simulink model "UPQC_model"  (R2020b)
settings: Solver=FixedStepAuto  StartTime=0.0  StopTime=Tsim  FixedStep=Tsample  MaxStep=Tsample  RelTol=1e-3
values from neighbouring files (symbols this model uses):
  C_parallel_Series = zeros(1,4)    [Netzmodell_Ini_DL.m]    (also in workspace_Ini.mat = [1e-05 1e-05 1e-05 0])
  C_parallel_Shunt = zeros(1,4)    [Netzmodell_Ini_DL.m]    (also in workspace_Ini.mat = [1e-05 1e-05 1e-05 0])
  CC_Ki = 5    [Netzmodell_Ini_DL.m]    (also in workspace_Ini.mat)
  CC_Ki_geg = 5    [Netzmodell_Ini_DL.m]    (also in workspace_Ini.mat)
  CC_Kp = 10    [Netzmodell_Ini_DL.m]    (also in workspace_Ini.mat)
  CC_Kp_geg = 10    [Netzmodell_Ini_DL.m]    (also in workspace_Ini.mat)
  CC_OS =     [workspace_Ini.mat]
  Czk = Szenario.Czk*u    [Netzmodell_Ini_DL.m]    (also in workspace_Ini.mat = 0.003)
  fak_RVC = Szenario.fak_RVC    [Netzmodell_Ini_DL.m]    (also in workspace_Ini.mat = [1 1 1])
  fak_Uns = [1; 1; 1]    [Netzmodell_Ini_DL.m]    (also in workspace_Ini.mat = [1 1 1])
  Flicker_Schaltzeitpunkte_L1 = Schaltzeitpunkte(1,:)    [Netzmodell_Ini_DL.m]    (also in workspace_Ini.mat = 10.5)
  Flicker_Schaltzeitpunkte_L2 = Schaltzeitpunkte(2,:)    [Netzmodell_Ini_DL.m]    (also in workspace_Ini.mat = 10.5)
  Flicker_Schaltzeitpunkte_L3 = Schaltzeitpunkte(3,:)    [Netzmodell_Ini_DL.m]    (also in workspace_Ini.mat = 10.5)
  fs = [f_nom; f_nom; f_nom]    [Netzmodell_Ini_DL.m]    (also in workspace_Ini.mat = [50 50 50])
  fsw = Szenario.fsw*k    [Netzmodell_Ini_DL.m]    (also in workspace_Ini.mat = 20000)
  I_Basis_Ober_L1 = I_Basis_Ober(1)    [Netzmodell_Ini_DL.m]    (also in workspace_Ini.mat = 0)
  I_Basis_Ober_L2 = I_Basis_Ober(2)    [Netzmodell_Ini_DL.m]    (also in workspace_Ini.mat = 0)
  I_Basis_Ober_L3 = I_Basis_Ober(3)    [Netzmodell_Ini_DL.m]    (also in workspace_Ini.mat = 0)
  I_relativ_Ober_L1 = Szenario.I_relativ_Ober_L1    [Netzmodell_Ini_DL.m]    (also in workspace_Ini.mat = [0 100 0 100 100 0 100 100 0 0 0 0 ... (50 elements, 1x50)])
  I_relativ_Ober_L2 = Szenario.I_relativ_Ober_L2    [Netzmodell_Ini_DL.m]    (also in workspace_Ini.mat = [0 100 0 100 100 0 100 100 0 0 0 0 ... (50 elements, 1x50)])
  I_relativ_Ober_L3 = Szenario.I_relativ_Ober_L3    [Netzmodell_Ini_DL.m]    (also in workspace_Ini.mat = [0 100 0 100 100 0 100 100 0 0 0 0 ... (50 elements, 1x50)])
  L_Ausgang_Series = zeros(1,4)    [Netzmodell_Ini_DL.m]    (also in workspace_Ini.mat = [0.00093 0.00093 0.00093 0.00093])
  L_Ausgang_Shunt = zeros(1,4)    [Netzmodell_Ini_DL.m]    (also in workspace_Ini.mat = [0.00093 0.00093 0.00093 0.00093])
  L_Eingang_Series = zeros(1,4)    [Netzmodell_Ini_DL.m]    (also in workspace_Ini.mat = [0.00085 0.00085 0.00085 0.00085])
  L_Eingang_Shunt = zeros(1,4)    [Netzmodell_Ini_DL.m]    (also in workspace_Ini.mat = [0.00085 0.00085 0.00085 0.00085])
  Ls_in = 52.2*u/10    (= 5.22e-06)    [Netzmodell_Ini_DL.m]    (also in workspace_Ini.mat)
  Ltrans = Szenario.Ltrans*m    [Netzmodell_Ini_DL.m]    (also in workspace_Ini.mat = 0.000256)
  OS_off = 6    [Netzmodell_Ini_DL.m]    (also in workspace_Ini.mat)
  OS_on = 1    [Netzmodell_Ini_DL.m]    (also in workspace_Ini.mat)
  Phi_Ober_L1 = Phi_Ober(1)    [Netzmodell_Ini_DL.m]    (also in workspace_Ini.mat = 0)
  Phi_Ober_L2 = Phi_Ober(2)    [Netzmodell_Ini_DL.m]    (also in workspace_Ini.mat = -120)
  Phi_Ober_L3 = Phi_Ober(3)    [Netzmodell_Ini_DL.m]    (also in workspace_Ini.mat = 120)
  Phis = [0; -120; 120]    [Netzmodell_Ini_DL.m]    (also in workspace_Ini.mat = [0 -120 120])
  Pl_Flicker = Pl_Flicker*k    [Netzmodell_Ini_DL.m]    (also in workspace_Ini.mat = [5000 5000 5000])
  Pl_Grund = Szenario.Pl_Grund *k    [Netzmodell_Ini_DL.m]    (also in workspace_Ini.mat = [5 5 5])
  Pl_RVC = Pl_RVC*k    [Netzmodell_Ini_DL.m]    (also in workspace_Ini.mat = [10000 10000 10000])
  Pl_Uns = Pl_Uns*k    [Netzmodell_Ini_DL.m]    (also in workspace_Ini.mat = [25000 10 10])
  Ql_ind_Flicker = Ql_ind_Flicker*k    [Netzmodell_Ini_DL.m]    (also in workspace_Ini.mat = [0 0 0])
  Ql_ind_Grund = Szenario.Ql_ind_Grund*k    [Netzmodell_Ini_DL.m]    (also in workspace_Ini.mat = [0 0 0])
  Ql_ind_RVC = Szenario.Ql_ind_RVC*k    [Netzmodell_Ini_DL.m]    (also in workspace_Ini.mat = [0 0 0])
  Ql_ind_Uns = Ql_ind_Uns*k    [Netzmodell_Ini_DL.m]    (also in workspace_Ini.mat = [0 0 0])
  Ql_kap_Flicker = Ql_kap_Flicker*k    [Netzmodell_Ini_DL.m]    (also in workspace_Ini.mat = [0 0 0])
  Ql_kap_Grund = Szenario.Ql_kap_Grund*k    [Netzmodell_Ini_DL.m]    (also in workspace_Ini.mat = [0 0 0])
  Ql_kap_RVC = Szenario.Ql_kap_RVC*k    [Netzmodell_Ini_DL.m]    (also in workspace_Ini.mat = [0 0 0])
  Ql_kap_Uns = Ql_kap_Uns*k    [Netzmodell_Ini_DL.m]    (also in workspace_Ini.mat = [0 0 0])
  R_Ausgang_Series = zeros(1,4)    [Netzmodell_Ini_DL.m]    (also in workspace_Ini.mat = [0.1 0.1 0.1 0.1])
  R_Ausgang_Shunt = zeros(1,4)    [Netzmodell_Ini_DL.m]    (also in workspace_Ini.mat = [0.1 0.1 0.1 0.1])
  R_Eingang_Series = zeros(1,4)    [Netzmodell_Ini_DL.m]    (also in workspace_Ini.mat = [0.1 0.1 0.1 0.1])
  R_Eingang_Shunt = zeros(1,4)    [Netzmodell_Ini_DL.m]    (also in workspace_Ini.mat = [0.1 0.1 0.1 0.1])
  R_parallel_Series = zeros(1,4)    [Netzmodell_Ini_DL.m]    (also in workspace_Ini.mat = [13 13 13 0])
  R_parallel_Shunt = zeros(1,4)    [Netzmodell_Ini_DL.m]    (also in workspace_Ini.mat = [13 13 13 0])
  R_ZK_Belastung = 20    [Netzmodell_Ini_DL.m]    (also in workspace_Ini.mat)
  Rs_in = 5.2*m/10    (= 0.00052)    [Netzmodell_Ini_DL.m]    (also in workspace_Ini.mat)
  Rtrans = Szenario.Rtrans    [Netzmodell_Ini_DL.m]    (also in workspace_Ini.mat = 0.206)
  RVC_L1_on_off_Zeitpunkte = Szenario.RVC_L1_on_off_Zeitpunkte    [Netzmodell_Ini_DL.m]    (also in workspace_Ini.mat = [10.5 40 10 11 12 13 14 15])
  RVC_L2_on_off_Zeitpunkte = Szenario.RVC_L2_on_off_Zeitpunkte    [Netzmodell_Ini_DL.m]    (also in workspace_Ini.mat = [10.5 40 10 11 12 13 14 15])
  RVC_L3_on_off_Zeitpunkte = Szenario.RVC_L3_on_off_Zeitpunkte    [Netzmodell_Ini_DL.m]    (also in workspace_Ini.mat = [10.5 40 10 11 12 13 14 15])
  RVC_off = 20.5    [Netzmodell_Ini_DL.m]    (also in workspace_Ini.mat)
  RVC_on = 20    [Netzmodell_Ini_DL.m]    (also in workspace_Ini.mat)
  RVC_val = [0.8,0.8,0.8]    [Netzmodell_Ini_DL.m]    (also in workspace_Ini.mat = [0.8 0.8 0.8])
  strans = Szenario.strans    [Netzmodell_Ini_DL.m]    (also in workspace_Ini.mat = 0.25)
  t_breaker_series = tacts    [Netzmodell_Ini_DL.m]    (also in workspace_Ini.mat = 0.5)
  tact = Szenario.tact    [Netzmodell_Ini_DL.m]    (also in workspace_Ini.mat = 0.5)
  tact_OS_Regler = Szenario.tact_OS_Regler    [Netzmodell_Ini_DL.m]    (also in workspace_Ini.mat = 0.5)
  tact_QU = 10    [Netzmodell_Ini_DL.m]    (also in workspace_Ini.mat)
  tacts = Szenario.tacts    [Netzmodell_Ini_DL.m]    (also in workspace_Ini.mat = 0.5)
  Tsample = Szenario.Tsample    [Netzmodell_Ini_DL.m]    (also in workspace_Ini.mat = 5e-06)
  Uns_L1_on_off_Zeitpunkte = Szenario.Uns_L1_on_off_Zeitpunkte    [Netzmodell_Ini_DL.m]    (also in workspace_Ini.mat = [1 6 10 11 12 13 14 15])
  Uns_L2_on_off_Zeitpunkte = Szenario.Uns_L2_on_off_Zeitpunkte    [Netzmodell_Ini_DL.m]    (also in workspace_Ini.mat = [10 30 10 11 12 13 14 15])
  Uns_L3_on_off_Zeitpunkte = Szenario.Uns_L3_on_off_Zeitpunkte    [Netzmodell_Ini_DL.m]    (also in workspace_Ini.mat = [10 30 10 11 12 13 14 15])
  Us = [Us_Amp; Us_Amp; Us_Amp]    [Netzmodell_Ini_DL.m]    (also in workspace_Ini.mat = [326.598632371 326.598632371 326.598632371])
  Us_Amp = sqrt(2)*400/sqrt(3)    [Netzmodell_Ini_DL.m]    (also in workspace_Ini.mat = 326.598632371)
  VC_Ki_gegen = 30    [Netzmodell_Ini_DL.m]    (also in workspace_Ini.mat)
  VC_Ki_gegen_shunt = 15    [Netzmodell_Ini_DL.m]    (also in workspace_Ini.mat)
  VC_Ki_mit = 5    [Netzmodell_Ini_DL.m]    (also in workspace_Ini.mat)
  VC_Kp_gegen = 5    [workspace_Ini.mat]
  VC_Kp_gegen_shunt = 2    [Netzmodell_Ini_DL.m]    (also in workspace_Ini.mat)
  VC_Kp_mit = 10    [Netzmodell_Ini_DL.m]    (also in workspace_Ini.mat)
  VC_ZK_Ki = 5    [Netzmodell_Ini_DL.m]    (also in workspace_Ini.mat)
  VC_ZK_Kp = 0.5    [Netzmodell_Ini_DL.m]    (also in workspace_Ini.mat)
  Vielfache_Ober_L1 = Szenario.Vielfache_Ober_L1    [Netzmodell_Ini_DL.m]    (also in workspace_Ini.mat = [1 2 3 4 5 6 7 8 9 10 11 12 ... (50 elements, 1x50)])
  Vielfache_Ober_L2 = Szenario.Vielfache_Ober_L2    [Netzmodell_Ini_DL.m]    (also in workspace_Ini.mat = [1 2 3 4 5 6 7 8 9 10 11 12 ... (50 elements, 1x50)])
  Vielfache_Ober_L3 = Szenario.Vielfache_Ober_L3    [Netzmodell_Ini_DL.m]    (also in workspace_Ini.mat = [1 2 3 4 5 6 7 8 9 10 11 12 ... (50 elements, 1x50)])
  ZK_Belastung_off = 100    [Netzmodell_Ini_DL.m]    (also in workspace_Ini.mat)
  ZK_Belastung_on = 100    [Netzmodell_Ini_DL.m]    (also in workspace_Ini.mat)
  Zwischenkreisspannung = 700    [Netzmodell_Ini_DL.m]    (also in workspace_Ini.mat)
undefined symbols (not defined in the file or in its folder): LAusgang, RReiheL3
libraries: powerlib x221, powerlib_meascontrol x80, pid_lib x23, eeTransforms x4, eePwmGeneratorTwoLevel x2, dspstat3 x1
(part 15 of 16)

== system UPQC_model/Shunt UPQC/Shuntkompensator/dq_Netz/Tdq+1_4 ==
  In1 : Inport
  In2 : Inport  Port=2
  Add : Sum  Inputs=|++
  Add1 : Sum  Inputs=|++
  Cos : Trigonometry  Operator=cos
  Cos1 : Trigonometry  Operator=cos
  Demux : Demux  Outputs=2
  Gain : Gain  Gain=-1
  Mux : Mux  Inputs=2
  Product{,1..3} (4 alike) : Product
  Sin : Trigonometry
  Sin1 : Trigonometry
  Out1 : Outport
  wires:
  Add1/1 -> Mux/2
  Product3/1 -> Add1/2
  [alpha] -> Product2/1
  [alpha] -> Product/1
  Product/1 -> Add/1
  Cos1/1 -> Product3/1
  Sin1/1 -> Gain/1
  [beta] -> Product1/2
  Product1/1 -> Add/2
  Gain/1 -> Product2/2
  Mux/1 -> [dq]
  Add/1 -> Mux/1
  Sin/1 -> Product1/1
  Product2/1 -> Add1/1
  [beta] -> Product3/2
  Cos/1 -> Product/2
  In1/1 -> Demux/1  "vab"
  [dq] -> Out1/1  "dq"
  In2/1 -> [theta]  "theta"
  [theta] -> Sin/1, Cos/1
  [theta] -> Sin1/1, Cos1/1
  Demux/1 -> [alpha]
  Demux/2 -> [beta]

== system UPQC_model/Shunt UPQC/Shuntkompensator/dq_Netz/Tdq+1_5 ==
  In1 : Inport
  In2 : Inport  Port=2
  Add : Sum  Inputs=|++
  Add1 : Sum  Inputs=|++
  Cos : Trigonometry  Operator=cos
  Cos1 : Trigonometry  Operator=cos
  Demux : Demux  Outputs=2
  Gain : Gain  Gain=-1
  Mux : Mux  Inputs=2
  Product{,1..3} (4 alike) : Product
  Sin : Trigonometry
  Sin1 : Trigonometry
  Out1 : Outport
  wires:
  Add1/1 -> Mux/2
  Product3/1 -> Add1/2
  [alpha] -> Product2/1
  [alpha] -> Product/1
  Product/1 -> Add/1
  Cos1/1 -> Product3/1
  Sin1/1 -> Gain/1
  [beta] -> Product1/2
  Product1/1 -> Add/2
  Gain/1 -> Product2/2
  Mux/1 -> [dq]
  Add/1 -> Mux/1
  Sin/1 -> Product1/1
  Product2/1 -> Add1/1
  [beta] -> Product3/2
  Cos/1 -> Product/2
  In1/1 -> Demux/1  "vab"
  [dq] -> Out1/1  "dq"
  In2/1 -> [theta]  "theta"
  [theta] -> Sin/1, Cos/1
  [theta] -> Sin1/1, Cos1/1
  Demux/1 -> [alpha]
  Demux/2 -> [beta]

== system UPQC_model/Shunt UPQC/Shuntkompensator/dq_Netz/Tdq+1_6 ==
  In1 : Inport
  In2 : Inport  Port=2
  Add : Sum  Inputs=|++
  Add1 : Sum  Inputs=|++
  Cos : Trigonometry  Operator=cos
  Cos1 : Trigonometry  Operator=cos
  Demux : Demux  Outputs=2
  Gain : Gain  Gain=-1
  Mux : Mux  Inputs=2
  Product{,1..3} (4 alike) : Product
  Sin : Trigonometry
  Sin1 : Trigonometry
  Out1 : Outport
  wires:
  Demux/2 -> [beta]
  Demux/1 -> [alpha]
  [theta] -> Cos1/1, Sin1/1
  [theta] -> Cos/1, Sin/1
  In2/1 -> [theta]  "theta"
  [dq] -> Out1/1  "dq"
  In1/1 -> Demux/1  "vab"
  Cos/1 -> Product/2
  [beta] -> Product3/2
  Product2/1 -> Add1/1
  Sin/1 -> Product1/1
  Add/1 -> Mux/1
  Mux/1 -> [dq]
  Gain/1 -> Product2/2
  Product1/1 -> Add/2
  [beta] -> Product1/2
  Sin1/1 -> Gain/1
  Cos1/1 -> Product3/1
  Product/1 -> Add/1
  [alpha] -> Product/1
  [alpha] -> Product2/1
  Product3/1 -> Add1/2
  Add1/1 -> Mux/2

== system UPQC_model/Shunt UPQC/Shuntkompensator/dq_Netz/Tdq+1_7 ==
  In1 : Inport
  In2 : Inport  Port=2
  Add : Sum  Inputs=|++
  Add1 : Sum  Inputs=|++
  Cos : Trigonometry  Operator=cos
  Cos1 : Trigonometry  Operator=cos
  Demux : Demux  Outputs=2
  Gain : Gain  Gain=-1
  Mux : Mux  Inputs=2
  Product{,1..3} (4 alike) : Product
  Sin : Trigonometry
  Sin1 : Trigonometry
  Out1 : Outport
  wires:
  Add1/1 -> Mux/2
  Product3/1 -> Add1/2
  [alpha] -> Product2/1
  [alpha] -> Product/1
  Product/1 -> Add/1
  Cos1/1 -> Product3/1
  Sin1/1 -> Gain/1
  [beta] -> Product1/2
  Product1/1 -> Add/2
  Gain/1 -> Product2/2
  Mux/1 -> [dq]
  Add/1 -> Mux/1
  Sin/1 -> Product1/1
  Product2/1 -> Add1/1
  [beta] -> Product3/2
  Cos/1 -> Product/2
  In1/1 -> Demux/1  "vab"
  [dq] -> Out1/1  "dq"
  In2/1 -> [theta]  "theta"
  [theta] -> Sin/1, Cos/1
  [theta] -> Sin1/1, Cos1/1
  Demux/1 -> [alpha]
  Demux/2 -> [beta]

== system UPQC_model/Shunt UPQC/Shuntkompensator/dq_Netz/Tdq+1_8 ==
  In1 : Inport
  In2 : Inport  Port=2
  Add : Sum  Inputs=|++
  Add1 : Sum  Inputs=|++
  Cos : Trigonometry  Operator=cos
  Cos1 : Trigonometry  Operator=cos
  Demux : Demux  Outputs=2
  Gain : Gain  Gain=-1
  Mux : Mux  Inputs=2
  Product{,1..3} (4 alike) : Product
  Sin : Trigonometry
  Sin1 : Trigonometry
  Out1 : Outport
  wires:
  Demux/2 -> [beta]
  Demux/1 -> [alpha]
  [theta] -> Cos1/1, Sin1/1
  [theta] -> Cos/1, Sin/1
  In2/1 -> [theta]  "theta"
  [dq] -> Out1/1  "dq"
  In1/1 -> Demux/1  "vab"
  Cos/1 -> Product/2
  [beta] -> Product3/2
  Product2/1 -> Add1/1
  Sin/1 -> Product1/1
  Add/1 -> Mux/1
  Mux/1 -> [dq]
  Gain/1 -> Product2/2
  Product1/1 -> Add/2
  [beta] -> Product1/2
  Sin1/1 -> Gain/1
  Cos1/1 -> Product3/1
  Product/1 -> Add/1
  [alpha] -> Product/1
  [alpha] -> Product2/1
  Product3/1 -> Add1/2
  Add1/1 -> Mux/2

== system UPQC_model/Shunt UPQC/Shuntkompensator/dq_Shunt/Entkopplungszelle1 ==
  In3 : Inport
  In4 : Inport  Port=2
  In1 : Inport  Port=3
  Add : Sum  Inputs=|+-
  Add1 : Sum  Inputs=|+-
  Add2 : Sum  Inputs=|++
  Add3 : Sum  Inputs=|+-
  Cos : Trigonometry  Operator=cos
  Demux : Demux  Outputs=2
  Demux1 : Demux  Outputs=2
  Mux : Mux  Inputs=2
  Product{,1..3} (4 alike) : Product
  Sin : Trigonometry
  Out2 : Outport
  wires:
  Mux/1 -> Out2/1
  Demux1/1 -> Product1/1, Product/2  "d"
  In1/1 -> Demux1/1  "dq"
  In4/1 -> Sin/1, Cos/1  "theta"
  Add3/1 -> Mux/2
  Add1/1 -> Mux/1
  Product1/1 -> Add2/2
  Product2/1 -> Add3/2
  In3/1 -> Demux/1  "vdqmit"
  Sin/1 -> Product1/2, Product3/1
  Cos/1 -> Product2/2, Product/1
  Add/1 -> Add1/1
  Demux/2 -> Add2/1
  Product3/1 -> Add1/2
  Add2/1 -> Add3/1
  Demux/1 -> Add/1
  Demux1/2 -> Product3/2, Product2/1  "q"
  Product/1 -> Add/2

== system UPQC_model/Shunt UPQC/Shuntkompensator/dq_Shunt/Entkopplungszelle10 ==
  In3 : Inport
  In4 : Inport  Port=2
  In1 : Inport  Port=3
  Add : Sum  Inputs=|+-
  Add1 : Sum  Inputs=|+-
  Add2 : Sum  Inputs=|++
  Add3 : Sum  Inputs=|+-
  Cos : Trigonometry  Operator=cos
  Demux : Demux  Outputs=2
  Demux1 : Demux  Outputs=2
  Mux : Mux  Inputs=2
  Product{,1..3} (4 alike) : Product
  Sin : Trigonometry
  Out2 : Outport
  wires:
  Mux/1 -> Out2/1
  Demux1/1 -> Product1/1, Product/2  "d"
  In1/1 -> Demux1/1  "dq"
  In4/1 -> Sin/1, Cos/1  "theta"
  Add3/1 -> Mux/2
  Add1/1 -> Mux/1
  Product1/1 -> Add2/2
  Product2/1 -> Add3/2
  In3/1 -> Demux/1  "vdqmit"
  Sin/1 -> Product1/2, Product3/1
  Cos/1 -> Product2/2, Product/1
  Add/1 -> Add1/1
  Demux/2 -> Add2/1
  Product3/1 -> Add1/2
  Add2/1 -> Add3/1
  Demux/1 -> Add/1
  Demux1/2 -> Product3/2, Product2/1  "q"
  Product/1 -> Add/2

== system UPQC_model/Shunt UPQC/Shuntkompensator/dq_Shunt/Entkopplungszelle11 ==
  In3 : Inport
  In4 : Inport  Port=2
  In1 : Inport  Port=3
  Add : Sum  Inputs=|+-
  Add1 : Sum  Inputs=|+-
  Add2 : Sum  Inputs=|++
  Add3 : Sum  Inputs=|+-
  Cos : Trigonometry  Operator=cos
  Demux : Demux  Outputs=2
  Demux1 : Demux  Outputs=2
  Mux : Mux  Inputs=2
  Product{,1..3} (4 alike) : Product
  Sin : Trigonometry
  Out2 : Outport
  wires:
  Mux/1 -> Out2/1
  Demux1/1 -> Product1/1, Product/2  "d"
  In1/1 -> Demux1/1  "dq"
  In4/1 -> Sin/1, Cos/1  "theta"
  Add3/1 -> Mux/2
  Add1/1 -> Mux/1
  Product1/1 -> Add2/2
  Product2/1 -> Add3/2
  In3/1 -> Demux/1  "vdqmit"
  Sin/1 -> Product1/2, Product3/1
  Cos/1 -> Product2/2, Product/1
  Add/1 -> Add1/1
  Demux/2 -> Add2/1
  Product3/1 -> Add1/2
  Add2/1 -> Add3/1
  Demux/1 -> Add/1
  Demux1/2 -> Product3/2, Product2/1  "q"
  Product/1 -> Add/2

== system UPQC_model/Shunt UPQC/Shuntkompensator/dq_Shunt/Entkopplungszelle12 ==
  In3 : Inport
  In4 : Inport  Port=2
  In1 : Inport  Port=3
  Add : Sum  Inputs=|+-
  Add1 : Sum  Inputs=|+-
  Add2 : Sum  Inputs=|++
  Add3 : Sum  Inputs=|+-
  Cos : Trigonometry  Operator=cos
  Demux : Demux  Outputs=2
  Demux1 : Demux  Outputs=2
  Mux : Mux  Inputs=2
  Product{,1..3} (4 alike) : Product
  Sin : Trigonometry
  Out2 : Outport
  wires:
  Mux/1 -> Out2/1
  Demux1/1 -> Product1/1, Product/2  "d"
  In1/1 -> Demux1/1  "dq"
  In4/1 -> Sin/1, Cos/1  "theta"
  Add3/1 -> Mux/2
  Add1/1 -> Mux/1
  Product1/1 -> Add2/2
  Product2/1 -> Add3/2
  In3/1 -> Demux/1  "vdqmit"
  Sin/1 -> Product1/2, Product3/1
  Cos/1 -> Product2/2, Product/1
  Add/1 -> Add1/1
  Demux/2 -> Add2/1
  Product3/1 -> Add1/2
  Add2/1 -> Add3/1
  Demux/1 -> Add/1
  Demux1/2 -> Product3/2, Product2/1  "q"
  Product/1 -> Add/2

== system UPQC_model/Shunt UPQC/Shuntkompensator/dq_Shunt/Entkopplungszelle13 ==
  In3 : Inport
  In4 : Inport  Port=2
  In1 : Inport  Port=3
  Add : Sum  Inputs=|+-
  Add1 : Sum  Inputs=|+-
  Add2 : Sum  Inputs=|++
  Add3 : Sum  Inputs=|+-
  Cos : Trigonometry  Operator=cos
  Demux : Demux  Outputs=2
  Demux1 : Demux  Outputs=2
  Mux : Mux  Inputs=2
  Product{,1..3} (4 alike) : Product
  Sin : Trigonometry
  Out2 : Outport
  wires:
  Mux/1 -> Out2/1
  Demux1/1 -> Product1/1, Product/2  "d"
  In1/1 -> Demux1/1  "dq"
  In4/1 -> Sin/1, Cos/1  "theta"
  Add3/1 -> Mux/2
  Add1/1 -> Mux/1
  Product1/1 -> Add2/2
  Product2/1 -> Add3/2
  In3/1 -> Demux/1  "vdqmit"
  Sin/1 -> Product1/2, Product3/1
  Cos/1 -> Product2/2, Product/1
  Add/1 -> Add1/1
  Demux/2 -> Add2/1
  Product3/1 -> Add1/2
  Add2/1 -> Add3/1
  Demux/1 -> Add/1
  Demux1/2 -> Product3/2, Product2/1  "q"
  Product/1 -> Add/2

== system UPQC_model/Shunt UPQC/Shuntkompensator/dq_Shunt/Entkopplungszelle14 ==
  In3 : Inport
  In4 : Inport  Port=2
  In1 : Inport  Port=3
  Add : Sum  Inputs=|+-
  Add1 : Sum  Inputs=|+-
  Add2 : Sum  Inputs=|++
  Add3 : Sum  Inputs=|+-
  Cos : Trigonometry  Operator=cos
  Demux : Demux  Outputs=2
  Demux1 : Demux  Outputs=2
  Mux : Mux  Inputs=2
  Product{,1..3} (4 alike) : Product
  Sin : Trigonometry
  Out2 : Outport
  wires:
  Mux/1 -> Out2/1
  Demux1/1 -> Product1/1, Product/2  "d"
  In1/1 -> Demux1/1  "dq"
  In4/1 -> Sin/1, Cos/1  "theta"
  Add3/1 -> Mux/2
  Add1/1 -> Mux/1
  Product1/1 -> Add2/2
  Product2/1 -> Add3/2
  In3/1 -> Demux/1  "vdqmit"
  Sin/1 -> Product1/2, Product3/1
  Cos/1 -> Product2/2, Product/1
  Add/1 -> Add1/1
  Demux/2 -> Add2/1
  Product3/1 -> Add1/2
  Add2/1 -> Add3/1
  Demux/1 -> Add/1
  Demux1/2 -> Product3/2, Product2/1  "q"
  Product/1 -> Add/2

== system UPQC_model/Shunt UPQC/Shuntkompensator/dq_Shunt/Entkopplungszelle15 ==
  In3 : Inport
  In4 : Inport  Port=2
  In1 : Inport  Port=3
  Add : Sum  Inputs=|+-
  Add1 : Sum  Inputs=|+-
  Add2 : Sum  Inputs=|++
  Add3 : Sum  Inputs=|+-
  Cos : Trigonometry  Operator=cos
  Demux : Demux  Outputs=2
  Demux1 : Demux  Outputs=2
  Mux : Mux  Inputs=2
  Product{,1..3} (4 alike) : Product
  Sin : Trigonometry
  Out2 : Outport
  wires:
  Product/1 -> Add/2
  Demux1/2 -> Product2/1, Product3/2  "q"
  Demux/1 -> Add/1
  Add2/1 -> Add3/1
  Product3/1 -> Add1/2
  Demux/2 -> Add2/1
  Add/1 -> Add1/1
  Cos/1 -> Product/1, Product2/2
  Sin/1 -> Product3/1, Product1/2
  In3/1 -> Demux/1  "vdqmit"
  Product2/1 -> Add3/2
  Product1/1 -> Add2/2
  Add1/1 -> Mux/1
  Add3/1 -> Mux/2
  In4/1 -> Cos/1, Sin/1  "theta"
  In1/1 -> Demux1/1  "dq"
  Demux1/1 -> Product/2, Product1/1  "d"
  Mux/1 -> Out2/1

== system UPQC_model/Shunt UPQC/Shuntkompensator/dq_Shunt/Entkopplungszelle16 ==
  In3 : Inport
  In4 : Inport  Port=2
  In1 : Inport  Port=3
  Add : Sum  Inputs=|+-
  Add1 : Sum  Inputs=|+-
  Add2 : Sum  Inputs=|++
  Add3 : Sum  Inputs=|+-
  Cos : Trigonometry  Operator=cos
  Demux : Demux  Outputs=2
  Demux1 : Demux  Outputs=2
  Mux : Mux  Inputs=2
  Product{,1..3} (4 alike) : Product
  Sin : Trigonometry
  Out2 : Outport
  wires:
  Mux/1 -> Out2/1
  Demux1/1 -> Product1/1, Product/2  "d"
  In1/1 -> Demux1/1  "dq"
  In4/1 -> Sin/1, Cos/1  "theta"
  Add3/1 -> Mux/2
  Add1/1 -> Mux/1
  Product1/1 -> Add2/2
  Product2/1 -> Add3/2
  In3/1 -> Demux/1  "vdqmit"
  Sin/1 -> Product1/2, Product3/1
  Cos/1 -> Product2/2, Product/1
  Add/1 -> Add1/1
  Demux/2 -> Add2/1
  Product3/1 -> Add1/2
  Add2/1 -> Add3/1
  Demux/1 -> Add/1
  Demux1/2 -> Product3/2, Product2/1  "q"
  Product/1 -> Add/2

== system UPQC_model/Shunt UPQC/Shuntkompensator/dq_Shunt/Entkopplungszelle17 ==
  In3 : Inport
  In4 : Inport  Port=2
  In1 : Inport  Port=3
  Add : Sum  Inputs=|+-
  Add1 : Sum  Inputs=|+-
  Add2 : Sum  Inputs=|++
  Add3 : Sum  Inputs=|+-
  Cos : Trigonometry  Operator=cos
  Demux : Demux  Outputs=2
  Demux1 : Demux  Outputs=2
  Mux : Mux  Inputs=2
  Product{,1..3} (4 alike) : Product
  Sin : Trigonometry
  Out2 : Outport
  wires:
  Product/1 -> Add/2
  Demux1/2 -> Product2/1, Product3/2  "q"
  Demux/1 -> Add/1
  Add2/1 -> Add3/1
  Product3/1 -> Add1/2
  Demux/2 -> Add2/1
  Add/1 -> Add1/1
  Cos/1 -> Product/1, Product2/2
  Sin/1 -> Product3/1, Product1/2
  In3/1 -> Demux/1  "vdqmit"
  Product2/1 -> Add3/2
  Product1/1 -> Add2/2
  Add1/1 -> Mux/1
  Add3/1 -> Mux/2
  In4/1 -> Cos/1, Sin/1  "theta"
  In1/1 -> Demux1/1  "dq"
  Demux1/1 -> Product/2, Product1/1  "d"
  Mux/1 -> Out2/1

== system UPQC_model/Shunt UPQC/Shuntkompensator/dq_Shunt/Entkopplungszelle18 ==
  In3 : Inport
  In4 : Inport  Port=2
  In1 : Inport  Port=3
  Add : Sum  Inputs=|+-
  Add1 : Sum  Inputs=|+-
  Add2 : Sum  Inputs=|++
  Add3 : Sum  Inputs=|+-
  Cos : Trigonometry  Operator=cos
  Demux : Demux  Outputs=2
  Demux1 : Demux  Outputs=2
  Mux : Mux  Inputs=2
  Product{,1..3} (4 alike) : Product
  Sin : Trigonometry
  Out2 : Outport
  wires:
  Mux/1 -> Out2/1
  Demux1/1 -> Product1/1, Product/2  "d"
  In1/1 -> Demux1/1  "dq"
  In4/1 -> Sin/1, Cos/1  "theta"
  Add3/1 -> Mux/2
  Add1/1 -> Mux/1
  Product1/1 -> Add2/2
  Product2/1 -> Add3/2
  In3/1 -> Demux/1  "vdqmit"
  Sin/1 -> Product1/2, Product3/1
  Cos/1 -> Product2/2, Product/1
  Add/1 -> Add1/1
  Demux/2 -> Add2/1
  Product3/1 -> Add1/2
  Add2/1 -> Add3/1
  Demux/1 -> Add/1
  Demux1/2 -> Product3/2, Product2/1  "q"
  Product/1 -> Add/2

== system UPQC_model/Shunt UPQC/Shuntkompensator/dq_Shunt/Entkopplungszelle19 ==
  In3 : Inport
  In4 : Inport  Port=2
  In1 : Inport  Port=3
  Add : Sum  Inputs=|+-
  Add1 : Sum  Inputs=|+-
  Add2 : Sum  Inputs=|++
  Add3 : Sum  Inputs=|+-
  Cos : Trigonometry  Operator=cos
  Demux : Demux  Outputs=2
  Demux1 : Demux  Outputs=2
  Mux : Mux  Inputs=2
  Product{,1..3} (4 alike) : Product
  Sin : Trigonometry
  Out2 : Outport
  wires:
  Product/1 -> Add/2
  Demux1/2 -> Product2/1, Product3/2  "q"
  Demux/1 -> Add/1
  Add2/1 -> Add3/1
  Product3/1 -> Add1/2
  Demux/2 -> Add2/1
  Add/1 -> Add1/1
  Cos/1 -> Product/1, Product2/2
  Sin/1 -> Product3/1, Product1/2
  In3/1 -> Demux/1  "vdqmit"
  Product2/1 -> Add3/2
  Product1/1 -> Add2/2
  Add1/1 -> Mux/1
  Add3/1 -> Mux/2
  In4/1 -> Cos/1, Sin/1  "theta"
  In1/1 -> Demux1/1  "dq"
  Demux1/1 -> Product/2, Product1/1  "d"
  Mux/1 -> Out2/1

== system UPQC_model/Shunt UPQC/Shuntkompensator/dq_Shunt/Entkopplungszelle2 ==
  In3 : Inport
  In4 : Inport  Port=2
  In1 : Inport  Port=3
  Add : Sum  Inputs=|+-
  Add1 : Sum  Inputs=|+-
  Add2 : Sum  Inputs=|++
  Add3 : Sum  Inputs=|+-
  Cos : Trigonometry  Operator=cos
  Demux : Demux  Outputs=2
  Demux1 : Demux  Outputs=2
  Mux : Mux  Inputs=2
  Product{,1..3} (4 alike) : Product
  Sin : Trigonometry
  Out2 : Outport
  wires:
  Mux/1 -> Out2/1
  Demux1/1 -> Product1/1, Product/2  "d"
  In1/1 -> Demux1/1  "dq"
  In4/1 -> Sin/1, Cos/1  "theta"
  Add3/1 -> Mux/2
  Add1/1 -> Mux/1
  Product1/1 -> Add2/2
  Product2/1 -> Add3/2
  In3/1 -> Demux/1  "vdqmit"
  Sin/1 -> Product1/2, Product3/1
  Cos/1 -> Product2/2, Product/1
  Add/1 -> Add1/1
  Demux/2 -> Add2/1
  Product3/1 -> Add1/2
  Add2/1 -> Add3/1
  Demux/1 -> Add/1
  Demux1/2 -> Product3/2, Product2/1  "q"
  Product/1 -> Add/2

== system UPQC_model/Shunt UPQC/Shuntkompensator/dq_Shunt/Entkopplungszelle20 ==
  In3 : Inport
  In4 : Inport  Port=2
  In1 : Inport  Port=3
  Add : Sum  Inputs=|+-
  Add1 : Sum  Inputs=|+-
  Add2 : Sum  Inputs=|++
  Add3 : Sum  Inputs=|+-
  Cos : Trigonometry  Operator=cos
  Demux : Demux  Outputs=2
  Demux1 : Demux  Outputs=2
  Mux : Mux  Inputs=2
  Product{,1..3} (4 alike) : Product
  Sin : Trigonometry
  Out2 : Outport
  wires:
  Mux/1 -> Out2/1
  Demux1/1 -> Product1/1, Product/2  "d"
  In1/1 -> Demux1/1  "dq"
  In4/1 -> Sin/1, Cos/1  "theta"
  Add3/1 -> Mux/2
  Add1/1 -> Mux/1
  Product1/1 -> Add2/2
  Product2/1 -> Add3/2
  In3/1 -> Demux/1  "vdqmit"
  Sin/1 -> Product1/2, Product3/1
  Cos/1 -> Product2/2, Product/1
  Add/1 -> Add1/1
  Demux/2 -> Add2/1
  Product3/1 -> Add1/2
  Add2/1 -> Add3/1
  Demux/1 -> Add/1
  Demux1/2 -> Product3/2, Product2/1  "q"
  Product/1 -> Add/2

== system UPQC_model/Shunt UPQC/Shuntkompensator/dq_Shunt/Entkopplungszelle21 ==
  In3 : Inport
  In4 : Inport  Port=2
  In1 : Inport  Port=3
  Add : Sum  Inputs=|+-
  Add1 : Sum  Inputs=|+-
  Add2 : Sum  Inputs=|++
  Add3 : Sum  Inputs=|+-
  Cos : Trigonometry  Operator=cos
  Demux : Demux  Outputs=2
  Demux1 : Demux  Outputs=2
  Mux : Mux  Inputs=2
  Product{,1..3} (4 alike) : Product
  Sin : Trigonometry
  Out2 : Outport
  wires:
  Product/1 -> Add/2
  Demux1/2 -> Product2/1, Product3/2  "q"
  Demux/1 -> Add/1
  Add2/1 -> Add3/1
  Product3/1 -> Add1/2
  Demux/2 -> Add2/1
  Add/1 -> Add1/1
  Cos/1 -> Product/1, Product2/2
  Sin/1 -> Product3/1, Product1/2
  In3/1 -> Demux/1  "vdqmit"
  Product2/1 -> Add3/2
  Product1/1 -> Add2/2
  Add1/1 -> Mux/1
  Add3/1 -> Mux/2
  In4/1 -> Cos/1, Sin/1  "theta"
  In1/1 -> Demux1/1  "dq"
  Demux1/1 -> Product/2, Product1/1  "d"
  Mux/1 -> Out2/1

== system UPQC_model/Shunt UPQC/Shuntkompensator/dq_Shunt/Entkopplungszelle22 ==
  In3 : Inport
  In4 : Inport  Port=2
  In1 : Inport  Port=3
  Add : Sum  Inputs=|+-
  Add1 : Sum  Inputs=|+-
  Add2 : Sum  Inputs=|++
  Add3 : Sum  Inputs=|+-
  Cos : Trigonometry  Operator=cos
  Demux : Demux  Outputs=2
  Demux1 : Demux  Outputs=2
  Mux : Mux  Inputs=2
  Product{,1..3} (4 alike) : Product
  Sin : Trigonometry
  Out2 : Outport
  wires:
  Mux/1 -> Out2/1
  Demux1/1 -> Product1/1, Product/2  "d"
  In1/1 -> Demux1/1  "dq"
  In4/1 -> Sin/1, Cos/1  "theta"
  Add3/1 -> Mux/2
  Add1/1 -> Mux/1
  Product1/1 -> Add2/2
  Product2/1 -> Add3/2
  In3/1 -> Demux/1  "vdqmit"
  Sin/1 -> Product1/2, Product3/1
  Cos/1 -> Product2/2, Product/1
  Add/1 -> Add1/1
  Demux/2 -> Add2/1
  Product3/1 -> Add1/2
  Add2/1 -> Add3/1
  Demux/1 -> Add/1
  Demux1/2 -> Product3/2, Product2/1  "q"
  Product/1 -> Add/2

== system UPQC_model/Shunt UPQC/Shuntkompensator/dq_Shunt/Entkopplungszelle23 ==
  In3 : Inport
  In4 : Inport  Port=2
  In1 : Inport  Port=3
  Add : Sum  Inputs=|+-
  Add1 : Sum  Inputs=|+-
  Add2 : Sum  Inputs=|++
  Add3 : Sum  Inputs=|+-
  Cos : Trigonometry  Operator=cos
  Demux : Demux  Outputs=2
  Demux1 : Demux  Outputs=2
  Mux : Mux  Inputs=2
  Product{,1..3} (4 alike) : Product
  Sin : Trigonometry
  Out2 : Outport
  wires:
  Product/1 -> Add/2
  Demux1/2 -> Product2/1, Product3/2  "q"
  Demux/1 -> Add/1
  Add2/1 -> Add3/1
  Product3/1 -> Add1/2
  Demux/2 -> Add2/1
  Add/1 -> Add1/1
  Cos/1 -> Product/1, Product2/2
  Sin/1 -> Product3/1, Product1/2
  In3/1 -> Demux/1  "vdqmit"
  Product2/1 -> Add3/2
  Product1/1 -> Add2/2
  Add1/1 -> Mux/1
  Add3/1 -> Mux/2
  In4/1 -> Cos/1, Sin/1  "theta"
  In1/1 -> Demux1/1  "dq"
  Demux1/1 -> Product/2, Product1/1  "d"
  Mux/1 -> Out2/1

== system UPQC_model/Shunt UPQC/Shuntkompensator/dq_Shunt/Entkopplungszelle24 ==
  In3 : Inport
  In4 : Inport  Port=2
  In1 : Inport  Port=3
  Add : Sum  Inputs=|+-
  Add1 : Sum  Inputs=|+-
  Add2 : Sum  Inputs=|++
  Add3 : Sum  Inputs=|+-
  Cos : Trigonometry  Operator=cos
  Demux : Demux  Outputs=2
  Demux1 : Demux  Outputs=2
  Mux : Mux  Inputs=2
  Product{,1..3} (4 alike) : Product
  Sin : Trigonometry
  Out2 : Outport
  wires:
  Mux/1 -> Out2/1
  Demux1/1 -> Product1/1, Product/2  "d"
  In1/1 -> Demux1/1  "dq"
  In4/1 -> Sin/1, Cos/1  "theta"
  Add3/1 -> Mux/2
  Add1/1 -> Mux/1
  Product1/1 -> Add2/2
  Product2/1 -> Add3/2
  In3/1 -> Demux/1  "vdqmit"
  Sin/1 -> Product1/2, Product3/1
  Cos/1 -> Product2/2, Product/1
  Add/1 -> Add1/1
  Demux/2 -> Add2/1
  Product3/1 -> Add1/2
  Add2/1 -> Add3/1
  Demux/1 -> Add/1
  Demux1/2 -> Product3/2, Product2/1  "q"
  Product/1 -> Add/2

== system UPQC_model/Shunt UPQC/Shuntkompensator/dq_Shunt/Entkopplungszelle25 ==
  In3 : Inport
  In4 : Inport  Port=2
  In1 : Inport  Port=3
  Add : Sum  Inputs=|+-
  Add1 : Sum  Inputs=|+-
  Add2 : Sum  Inputs=|++
  Add3 : Sum  Inputs=|+-
  Cos : Trigonometry  Operator=cos
  Demux : Demux  Outputs=2
  Demux1 : Demux  Outputs=2
  Mux : Mux  Inputs=2
  Product{,1..3} (4 alike) : Product
  Sin : Trigonometry
  Out2 : Outport
  wires:
  Product/1 -> Add/2
  Demux1/2 -> Product2/1, Product3/2  "q"
  Demux/1 -> Add/1
  Add2/1 -> Add3/1
  Product3/1 -> Add1/2
  Demux/2 -> Add2/1
  Add/1 -> Add1/1
  Cos/1 -> Product/1, Product2/2
  Sin/1 -> Product3/1, Product1/2
  In3/1 -> Demux/1  "vdqmit"
  Product2/1 -> Add3/2
  Product1/1 -> Add2/2
  Add1/1 -> Mux/1
  Add3/1 -> Mux/2
  In4/1 -> Cos/1, Sin/1  "theta"
  In1/1 -> Demux1/1  "dq"
  Demux1/1 -> Product/2, Product1/1  "d"
  Mux/1 -> Out2/1

== system UPQC_model/Shunt UPQC/Shuntkompensator/dq_Shunt/Entkopplungszelle26 ==
  In3 : Inport
  In4 : Inport  Port=2
  In1 : Inport  Port=3
  Add : Sum  Inputs=|+-
  Add1 : Sum  Inputs=|+-
  Add2 : Sum  Inputs=|++
  Add3 : Sum  Inputs=|+-
  Cos : Trigonometry  Operator=cos
  Demux : Demux  Outputs=2
  Demux1 : Demux  Outputs=2
  Mux : Mux  Inputs=2
  Product{,1..3} (4 alike) : Product
  Sin : Trigonometry
  Out2 : Outport
  wires:
  Mux/1 -> Out2/1
  Demux1/1 -> Product1/1, Product/2  "d"
  In1/1 -> Demux1/1  "dq"
  In4/1 -> Sin/1, Cos/1  "theta"
  Add3/1 -> Mux/2
  Add1/1 -> Mux/1
  Product1/1 -> Add2/2
  Product2/1 -> Add3/2
  In3/1 -> Demux/1  "vdqmit"
  Sin/1 -> Product1/2, Product3/1
  Cos/1 -> Product2/2, Product/1
  Add/1 -> Add1/1
  Demux/2 -> Add2/1
  Product3/1 -> Add1/2
  Add2/1 -> Add3/1
  Demux/1 -> Add/1
  Demux1/2 -> Product3/2, Product2/1  "q"
  Product/1 -> Add/2

== system UPQC_model/Shunt UPQC/Shuntkompensator/dq_Shunt/Entkopplungszelle27 ==
  In3 : Inport
  In4 : Inport  Port=2
  In1 : Inport  Port=3
  Add : Sum  Inputs=|+-
  Add1 : Sum  Inputs=|+-
  Add2 : Sum  Inputs=|++
  Add3 : Sum  Inputs=|+-
  Cos : Trigonometry  Operator=cos
  Demux : Demux  Outputs=2
  Demux1 : Demux  Outputs=2
  Mux : Mux  Inputs=2
  Product{,1..3} (4 alike) : Product
  Sin : Trigonometry
  Out2 : Outport
  wires:
  Product/1 -> Add/2
  Demux1/2 -> Product2/1, Product3/2  "q"
  Demux/1 -> Add/1
  Add2/1 -> Add3/1
  Product3/1 -> Add1/2
  Demux/2 -> Add2/1
  Add/1 -> Add1/1
  Cos/1 -> Product/1, Product2/2
  Sin/1 -> Product3/1, Product1/2
  In3/1 -> Demux/1  "vdqmit"
  Product2/1 -> Add3/2
  Product1/1 -> Add2/2
  Add1/1 -> Mux/1
  Add3/1 -> Mux/2
  In4/1 -> Cos/1, Sin/1  "theta"
  In1/1 -> Demux1/1  "dq"
  Demux1/1 -> Product/2, Product1/1  "d"
  Mux/1 -> Out2/1

== system UPQC_model/Shunt UPQC/Shuntkompensator/dq_Shunt/Entkopplungszelle28 ==
  In3 : Inport
  In4 : Inport  Port=2
  In1 : Inport  Port=3
  Add : Sum  Inputs=|+-
  Add1 : Sum  Inputs=|+-
  Add2 : Sum  Inputs=|++
  Add3 : Sum  Inputs=|+-
  Cos : Trigonometry  Operator=cos
  Demux : Demux  Outputs=2
  Demux1 : Demux  Outputs=2
  Mux : Mux  Inputs=2
  Product{,1..3} (4 alike) : Product
  Sin : Trigonometry
  Out2 : Outport
  wires:
  Product/1 -> Add/2
  Demux1/2 -> Product2/1, Product3/2  "q"
  Demux/1 -> Add/1
  Add2/1 -> Add3/1
  Product3/1 -> Add1/2
  Demux/2 -> Add2/1
  Add/1 -> Add1/1
  Cos/1 -> Product/1, Product2/2
  Sin/1 -> Product3/1, Product1/2
  In3/1 -> Demux/1  "vdqmit"
  Product2/1 -> Add3/2
  Product1/1 -> Add2/2
  Add1/1 -> Mux/1
  Add3/1 -> Mux/2
  In4/1 -> Cos/1, Sin/1  "theta"
  In1/1 -> Demux1/1  "dq"
  Demux1/1 -> Product/2, Product1/1  "d"
  Mux/1 -> Out2/1

== system UPQC_model/Shunt UPQC/Shuntkompensator/dq_Shunt/Entkopplungszelle29 ==
  In3 : Inport
  In4 : Inport  Port=2
  In1 : Inport  Port=3
  Add : Sum  Inputs=|+-
  Add1 : Sum  Inputs=|+-
  Add2 : Sum  Inputs=|++
  Add3 : Sum  Inputs=|+-
  Cos : Trigonometry  Operator=cos
  Demux : Demux  Outputs=2
  Demux1 : Demux  Outputs=2
  Mux : Mux  Inputs=2
  Product{,1..3} (4 alike) : Product
  Sin : Trigonometry
  Out2 : Outport
  wires:
  Product/1 -> Add/2
  Demux1/2 -> Product2/1, Product3/2  "q"
  Demux/1 -> Add/1
  Add2/1 -> Add3/1
  Product3/1 -> Add1/2
  Demux/2 -> Add2/1
  Add/1 -> Add1/1
  Cos/1 -> Product/1, Product2/2
  Sin/1 -> Product3/1, Product1/2
  In3/1 -> Demux/1  "vdqmit"
  Product2/1 -> Add3/2
  Product1/1 -> Add2/2
  Add1/1 -> Mux/1
  Add3/1 -> Mux/2
  In4/1 -> Cos/1, Sin/1  "theta"
  In1/1 -> Demux1/1  "dq"
  Demux1/1 -> Product/2, Product1/1  "d"
  Mux/1 -> Out2/1

== system UPQC_model/Shunt UPQC/Shuntkompensator/dq_Shunt/Entkopplungszelle3 ==
  In3 : Inport
  In4 : Inport  Port=2
  In1 : Inport  Port=3
  Add : Sum  Inputs=|+-
  Add1 : Sum  Inputs=|+-
  Add2 : Sum  Inputs=|++
  Add3 : Sum  Inputs=|+-
  Cos : Trigonometry  Operator=cos
  Demux : Demux  Outputs=2
  Demux1 : Demux  Outputs=2
  Mux : Mux  Inputs=2
  Product{,1..3} (4 alike) : Product
  Sin : Trigonometry
  Out2 : Outport
  wires:
  Mux/1 -> Out2/1
  Demux1/1 -> Product1/1, Product/2  "d"
  In1/1 -> Demux1/1  "dq"
  In4/1 -> Sin/1, Cos/1  "theta"
  Add3/1 -> Mux/2
  Add1/1 -> Mux/1
  Product1/1 -> Add2/2
  Product2/1 -> Add3/2
  In3/1 -> Demux/1  "vdqmit"
  Sin/1 -> Product1/2, Product3/1
  Cos/1 -> Product2/2, Product/1
  Add/1 -> Add1/1
  Demux/2 -> Add2/1
  Product3/1 -> Add1/2
  Add2/1 -> Add3/1
  Demux/1 -> Add/1
  Demux1/2 -> Product3/2, Product2/1  "q"
  Product/1 -> Add/2

== system UPQC_model/Shunt UPQC/Shuntkompensator/dq_Shunt/Entkopplungszelle30 ==
  In3 : Inport
  In4 : Inport  Port=2
  In1 : Inport  Port=3
  Add : Sum  Inputs=|+-
  Add1 : Sum  Inputs=|+-
  Add2 : Sum  Inputs=|++
  Add3 : Sum  Inputs=|+-
  Cos : Trigonometry  Operator=cos
  Demux : Demux  Outputs=2
  Demux1 : Demux  Outputs=2
  Mux : Mux  Inputs=2
  Product{,1..3} (4 alike) : Product
  Sin : Trigonometry
  Out2 : Outport
  wires:
  Product/1 -> Add/2
  Demux1/2 -> Product2/1, Product3/2  "q"
  Demux/1 -> Add/1
  Add2/1 -> Add3/1
  Product3/1 -> Add1/2
  Demux/2 -> Add2/1
  Add/1 -> Add1/1
  Cos/1 -> Product/1, Product2/2
  Sin/1 -> Product3/1, Product1/2
  In3/1 -> Demux/1  "vdqmit"
  Product2/1 -> Add3/2
  Product1/1 -> Add2/2
  Add1/1 -> Mux/1
  Add3/1 -> Mux/2
  In4/1 -> Cos/1, Sin/1  "theta"
  In1/1 -> Demux1/1  "dq"
  Demux1/1 -> Product/2, Product1/1  "d"
  Mux/1 -> Out2/1

== system UPQC_model/Shunt UPQC/Shuntkompensator/dq_Shunt/Entkopplungszelle31 ==
  In3 : Inport
  In4 : Inport  Port=2
  In1 : Inport  Port=3
  Add : Sum  Inputs=|+-
  Add1 : Sum  Inputs=|+-
  Add2 : Sum  Inputs=|++
  Add3 : Sum  Inputs=|+-
  Cos : Trigonometry  Operator=cos
  Demux : Demux  Outputs=2
  Demux1 : Demux  Outputs=2
  Mux : Mux  Inputs=2
  Product{,1..3} (4 alike) : Product
  Sin : Trigonometry
  Out2 : Outport
  wires:
  Mux/1 -> Out2/1
  Demux1/1 -> Product1/1, Product/2  "d"
  In1/1 -> Demux1/1  "dq"
  In4/1 -> Sin/1, Cos/1  "theta"
  Add3/1 -> Mux/2
  Add1/1 -> Mux/1
  Product1/1 -> Add2/2
  Product2/1 -> Add3/2
  In3/1 -> Demux/1  "vdqmit"
  Sin/1 -> Product1/2, Product3/1
  Cos/1 -> Product2/2, Product/1
  Add/1 -> Add1/1
  Demux/2 -> Add2/1
  Product3/1 -> Add1/2
  Add2/1 -> Add3/1
  Demux/1 -> Add/1
  Demux1/2 -> Product3/2, Product2/1  "q"
  Product/1 -> Add/2

== system UPQC_model/Shunt UPQC/Shuntkompensator/dq_Shunt/Entkopplungszelle32 ==
  In3 : Inport
  In4 : Inport  Port=2
  In1 : Inport  Port=3
  Add : Sum  Inputs=|+-
  Add1 : Sum  Inputs=|+-
  Add2 : Sum  Inputs=|++
  Add3 : Sum  Inputs=|+-
  Cos : Trigonometry  Operator=cos
  Demux : Demux  Outputs=2
  Demux1 : Demux  Outputs=2
  Mux : Mux  Inputs=2
  Product{,1..3} (4 alike) : Product
  Sin : Trigonometry
  Out2 : Outport
  wires:
  Product/1 -> Add/2
  Demux1/2 -> Product2/1, Product3/2  "q"
  Demux/1 -> Add/1
  Add2/1 -> Add3/1
  Product3/1 -> Add1/2
  Demux/2 -> Add2/1
  Add/1 -> Add1/1
  Cos/1 -> Product/1, Product2/2
  Sin/1 -> Product3/1, Product1/2
  In3/1 -> Demux/1  "vdqmit"
  Product2/1 -> Add3/2
  Product1/1 -> Add2/2
  Add1/1 -> Mux/1
  Add3/1 -> Mux/2
  In4/1 -> Cos/1, Sin/1  "theta"
  In1/1 -> Demux1/1  "dq"
  Demux1/1 -> Product/2, Product1/1  "d"
  Mux/1 -> Out2/1

== system UPQC_model/Shunt UPQC/Shuntkompensator/dq_Shunt/Entkopplungszelle33 ==
  In3 : Inport
  In4 : Inport  Port=2
  In1 : Inport  Port=3
  Add : Sum  Inputs=|+-
  Add1 : Sum  Inputs=|+-
  Add2 : Sum  Inputs=|++
  Add3 : Sum  Inputs=|+-
  Cos : Trigonometry  Operator=cos
  Demux : Demux  Outputs=2
  Demux1 : Demux  Outputs=2
  Mux : Mux  Inputs=2
  Product{,1..3} (4 alike) : Product
  Sin : Trigonometry
  Out2 : Outport
  wires:
  Product/1 -> Add/2
  Demux1/2 -> Product2/1, Product3/2  "q"
  Demux/1 -> Add/1
  Add2/1 -> Add3/1
  Product3/1 -> Add1/2
  Demux/2 -> Add2/1
  Add/1 -> Add1/1
  Cos/1 -> Product/1, Product2/2
  Sin/1 -> Product3/1, Product1/2
  In3/1 -> Demux/1  "vdqmit"
  Product2/1 -> Add3/2
  Product1/1 -> Add2/2
  Add1/1 -> Mux/1
  Add3/1 -> Mux/2
  In4/1 -> Cos/1, Sin/1  "theta"
  In1/1 -> Demux1/1  "dq"
  Demux1/1 -> Product/2, Product1/1  "d"
  Mux/1 -> Out2/1

== system UPQC_model/Shunt UPQC/Shuntkompensator/dq_Shunt/Entkopplungszelle34 ==
  In3 : Inport
  In4 : Inport  Port=2
  In1 : Inport  Port=3
  Add : Sum  Inputs=|+-
  Add1 : Sum  Inputs=|+-
  Add2 : Sum  Inputs=|++
  Add3 : Sum  Inputs=|+-
  Cos : Trigonometry  Operator=cos
  Demux : Demux  Outputs=2
  Demux1 : Demux  Outputs=2
  Mux : Mux  Inputs=2
  Product{,1..3} (4 alike) : Product
  Sin : Trigonometry
  Out2 : Outport
  wires:
  Mux/1 -> Out2/1
  Demux1/1 -> Product1/1, Product/2  "d"
  In1/1 -> Demux1/1  "dq"
  In4/1 -> Sin/1, Cos/1  "theta"
  Add3/1 -> Mux/2
  Add1/1 -> Mux/1
  Product1/1 -> Add2/2
  Product2/1 -> Add3/2
  In3/1 -> Demux/1  "vdqmit"
  Sin/1 -> Product1/2, Product3/1
  Cos/1 -> Product2/2, Product/1
  Add/1 -> Add1/1
  Demux/2 -> Add2/1
  Product3/1 -> Add1/2
  Add2/1 -> Add3/1
  Demux/1 -> Add/1
  Demux1/2 -> Product3/2, Product2/1  "q"
  Product/1 -> Add/2

== system UPQC_model/Shunt UPQC/Shuntkompensator/dq_Shunt/Entkopplungszelle35 ==
  In3 : Inport
  In4 : Inport  Port=2
  In1 : Inport  Port=3
  Add : Sum  Inputs=|+-
  Add1 : Sum  Inputs=|+-
  Add2 : Sum  Inputs=|++
  Add3 : Sum  Inputs=|+-
  Cos : Trigonometry  Operator=cos
  Demux : Demux  Outputs=2
  Demux1 : Demux  Outputs=2
  Mux : Mux  Inputs=2
  Product{,1..3} (4 alike) : Product
  Sin : Trigonometry
  Out2 : Outport
  wires:
  Product/1 -> Add/2
  Demux1/2 -> Product2/1, Product3/2  "q"
  Demux/1 -> Add/1
  Add2/1 -> Add3/1
  Product3/1 -> Add1/2
  Demux/2 -> Add2/1
  Add/1 -> Add1/1
  Cos/1 -> Product/1, Product2/2
  Sin/1 -> Product3/1, Product1/2
  In3/1 -> Demux/1  "vdqmit"
  Product2/1 -> Add3/2
  Product1/1 -> Add2/2
  Add1/1 -> Mux/1
  Add3/1 -> Mux/2
  In4/1 -> Cos/1, Sin/1  "theta"
  In1/1 -> Demux1/1  "dq"
  Demux1/1 -> Product/2, Product1/1  "d"
  Mux/1 -> Out2/1

== system UPQC_model/Shunt UPQC/Shuntkompensator/dq_Shunt/Entkopplungszelle36 ==
  In3 : Inport
  In4 : Inport  Port=2
  In1 : Inport  Port=3
  Add : Sum  Inputs=|+-
  Add1 : Sum  Inputs=|+-
  Add2 : Sum  Inputs=|++
  Add3 : Sum  Inputs=|+-
  Cos : Trigonometry  Operator=cos
  Demux : Demux  Outputs=2
  Demux1 : Demux  Outputs=2
  Mux : Mux  Inputs=2
  Product{,1..3} (4 alike) : Product
  Sin : Trigonometry
  Out2 : Outport
  wires:
  Product/1 -> Add/2
  Demux1/2 -> Product2/1, Product3/2  "q"
  Demux/1 -> Add/1
  Add2/1 -> Add3/1
  Product3/1 -> Add1/2
  Demux/2 -> Add2/1
  Add/1 -> Add1/1
  Cos/1 -> Product/1, Product2/2
  Sin/1 -> Product3/1, Product1/2
  In3/1 -> Demux/1  "vdqmit"
  Product2/1 -> Add3/2
  Product1/1 -> Add2/2
  Add1/1 -> Mux/1
  Add3/1 -> Mux/2
  In4/1 -> Cos/1, Sin/1  "theta"
  In1/1 -> Demux1/1  "dq"
  Demux1/1 -> Product/2, Product1/1  "d"
  Mux/1 -> Out2/1

== system UPQC_model/Shunt UPQC/Shuntkompensator/dq_Shunt/Entkopplungszelle37 ==
  In3 : Inport
  In4 : Inport  Port=2
  In1 : Inport  Port=3
  Add : Sum  Inputs=|+-
  Add1 : Sum  Inputs=|+-
  Add2 : Sum  Inputs=|++
  Add3 : Sum  Inputs=|+-
  Cos : Trigonometry  Operator=cos
  Demux : Demux  Outputs=2
  Demux1 : Demux  Outputs=2
  Mux : Mux  Inputs=2
  Product{,1..3} (4 alike) : Product
  Sin : Trigonometry
  Out2 : Outport
  wires:
  Mux/1 -> Out2/1
  Demux1/1 -> Product1/1, Product/2  "d"
  In1/1 -> Demux1/1  "dq"
  In4/1 -> Sin/1, Cos/1  "theta"
  Add3/1 -> Mux/2
  Add1/1 -> Mux/1
  Product1/1 -> Add2/2
  Product2/1 -> Add3/2
  In3/1 -> Demux/1  "vdqmit"
  Sin/1 -> Product1/2, Product3/1
  Cos/1 -> Product2/2, Product/1
  Add/1 -> Add1/1
  Demux/2 -> Add2/1
  Product3/1 -> Add1/2
  Add2/1 -> Add3/1
  Demux/1 -> Add/1
  Demux1/2 -> Product3/2, Product2/1  "q"
  Product/1 -> Add/2

== system UPQC_model/Shunt UPQC/Shuntkompensator/dq_Shunt/Entkopplungszelle38 ==
  In3 : Inport
  In4 : Inport  Port=2
  In1 : Inport  Port=3
  Add : Sum  Inputs=|+-
  Add1 : Sum  Inputs=|+-
  Add2 : Sum  Inputs=|++
  Add3 : Sum  Inputs=|+-
  Cos : Trigonometry  Operator=cos
  Demux : Demux  Outputs=2
  Demux1 : Demux  Outputs=2
  Mux : Mux  Inputs=2
  Product{,1..3} (4 alike) : Product
  Sin : Trigonometry
  Out2 : Outport
  wires:
  Product/1 -> Add/2
  Demux1/2 -> Product2/1, Product3/2  "q"
  Demux/1 -> Add/1
  Add2/1 -> Add3/1
  Product3/1 -> Add1/2
  Demux/2 -> Add2/1
  Add/1 -> Add1/1
  Cos/1 -> Product/1, Product2/2
  Sin/1 -> Product3/1, Product1/2
  In3/1 -> Demux/1  "vdqmit"
  Product2/1 -> Add3/2
  Product1/1 -> Add2/2
  Add1/1 -> Mux/1
  Add3/1 -> Mux/2
  In4/1 -> Cos/1, Sin/1  "theta"
  In1/1 -> Demux1/1  "dq"
  Demux1/1 -> Product/2, Product1/1  "d"
  Mux/1 -> Out2/1

== system UPQC_model/Shunt UPQC/Shuntkompensator/dq_Shunt/Entkopplungszelle39 ==
  In3 : Inport
  In4 : Inport  Port=2
  In1 : Inport  Port=3
  Add : Sum  Inputs=|+-
  Add1 : Sum  Inputs=|+-
  Add2 : Sum  Inputs=|++
  Add3 : Sum  Inputs=|+-
  Cos : Trigonometry  Operator=cos
  Demux : Demux  Outputs=2
  Demux1 : Demux  Outputs=2
  Mux : Mux  Inputs=2
  Product{,1..3} (4 alike) : Product
  Sin : Trigonometry
  Out2 : Outport
  wires:
  Mux/1 -> Out2/1
  Demux1/1 -> Product1/1, Product/2  "d"
  In1/1 -> Demux1/1  "dq"
  In4/1 -> Sin/1, Cos/1  "theta"
  Add3/1 -> Mux/2
  Add1/1 -> Mux/1
  Product1/1 -> Add2/2
  Product2/1 -> Add3/2
  In3/1 -> Demux/1  "vdqmit"
  Sin/1 -> Product1/2, Product3/1
  Cos/1 -> Product2/2, Product/1
  Add/1 -> Add1/1
  Demux/2 -> Add2/1
  Product3/1 -> Add1/2
  Add2/1 -> Add3/1
  Demux/1 -> Add/1
  Demux1/2 -> Product3/2, Product2/1  "q"
  Product/1 -> Add/2

== system UPQC_model/Shunt UPQC/Shuntkompensator/dq_Shunt/Entkopplungszelle4 ==
  In3 : Inport
  In4 : Inport  Port=2
  In1 : Inport  Port=3
  Add : Sum  Inputs=|+-
  Add1 : Sum  Inputs=|+-
  Add2 : Sum  Inputs=|++
  Add3 : Sum  Inputs=|+-
  Cos : Trigonometry  Operator=cos
  Demux : Demux  Outputs=2
  Demux1 : Demux  Outputs=2
  Mux : Mux  Inputs=2
  Product{,1..3} (4 alike) : Product
  Sin : Trigonometry
  Out2 : Outport
  wires:
  Mux/1 -> Out2/1
  Demux1/1 -> Product1/1, Product/2  "d"
  In1/1 -> Demux1/1  "dq"
  In4/1 -> Sin/1, Cos/1  "theta"
  Add3/1 -> Mux/2
  Add1/1 -> Mux/1
  Product1/1 -> Add2/2
  Product2/1 -> Add3/2
  In3/1 -> Demux/1  "vdqmit"
  Sin/1 -> Product1/2, Product3/1
  Cos/1 -> Product2/2, Product/1
  Add/1 -> Add1/1
  Demux/2 -> Add2/1
  Product3/1 -> Add1/2
  Add2/1 -> Add3/1
  Demux/1 -> Add/1
  Demux1/2 -> Product3/2, Product2/1  "q"
  Product/1 -> Add/2

== system UPQC_model/Shunt UPQC/Shuntkompensator/dq_Shunt/Entkopplungszelle40 ==
  In3 : Inport
  In4 : Inport  Port=2
  In1 : Inport  Port=3
  Add : Sum  Inputs=|+-
  Add1 : Sum  Inputs=|+-
  Add2 : Sum  Inputs=|++
  Add3 : Sum  Inputs=|+-
  Cos : Trigonometry  Operator=cos
  Demux : Demux  Outputs=2
  Demux1 : Demux  Outputs=2
  Mux : Mux  Inputs=2
  Product{,1..3} (4 alike) : Product
  Sin : Trigonometry
  Out2 : Outport
  wires:
  Product/1 -> Add/2
  Demux1/2 -> Product2/1, Product3/2  "q"
  Demux/1 -> Add/1
  Add2/1 -> Add3/1
  Product3/1 -> Add1/2
  Demux/2 -> Add2/1
  Add/1 -> Add1/1
  Cos/1 -> Product/1, Product2/2
  Sin/1 -> Product3/1, Product1/2
  In3/1 -> Demux/1  "vdqmit"
  Product2/1 -> Add3/2
  Product1/1 -> Add2/2
  Add1/1 -> Mux/1
  Add3/1 -> Mux/2
  In4/1 -> Cos/1, Sin/1  "theta"
  In1/1 -> Demux1/1  "dq"
  Demux1/1 -> Product/2, Product1/1  "d"
  Mux/1 -> Out2/1

== system UPQC_model/Shunt UPQC/Shuntkompensator/dq_Shunt/Entkopplungszelle41 ==
  In3 : Inport
  In4 : Inport  Port=2
  In1 : Inport  Port=3
  Add : Sum  Inputs=|+-
  Add1 : Sum  Inputs=|+-
  Add2 : Sum  Inputs=|++
  Add3 : Sum  Inputs=|+-
  Cos : Trigonometry  Operator=cos
  Demux : Demux  Outputs=2
  Demux1 : Demux  Outputs=2
  Mux : Mux  Inputs=2
  Product{,1..3} (4 alike) : Product
  Sin : Trigonometry
  Out2 : Outport
  wires:
  Mux/1 -> Out2/1
  Demux1/1 -> Product1/1, Product/2  "d"
  In1/1 -> Demux1/1  "dq"
  In4/1 -> Sin/1, Cos/1  "theta"
  Add3/1 -> Mux/2
  Add1/1 -> Mux/1
  Product1/1 -> Add2/2
  Product2/1 -> Add3/2
  In3/1 -> Demux/1  "vdqmit"
  Sin/1 -> Product1/2, Product3/1
  Cos/1 -> Product2/2, Product/1
  Add/1 -> Add1/1
  Demux/2 -> Add2/1
  Product3/1 -> Add1/2
  Add2/1 -> Add3/1
  Demux/1 -> Add/1
  Demux1/2 -> Product3/2, Product2/1  "q"
  Product/1 -> Add/2

== system UPQC_model/Shunt UPQC/Shuntkompensator/dq_Shunt/Entkopplungszelle42 ==
  In3 : Inport
  In4 : Inport  Port=2
  In1 : Inport  Port=3
  Add : Sum  Inputs=|+-
  Add1 : Sum  Inputs=|+-
  Add2 : Sum  Inputs=|++
  Add3 : Sum  Inputs=|+-
  Cos : Trigonometry  Operator=cos
  Demux : Demux  Outputs=2
  Demux1 : Demux  Outputs=2
  Mux : Mux  Inputs=2
  Product{,1..3} (4 alike) : Product
  Sin : Trigonometry
  Out2 : Outport
  wires:
  Mux/1 -> Out2/1
  Demux1/1 -> Product1/1, Product/2  "d"
  In1/1 -> Demux1/1  "dq"
  In4/1 -> Sin/1, Cos/1  "theta"
  Add3/1 -> Mux/2
  Add1/1 -> Mux/1
  Product1/1 -> Add2/2
  Product2/1 -> Add3/2
  In3/1 -> Demux/1  "vdqmit"
  Sin/1 -> Product1/2, Product3/1
  Cos/1 -> Product2/2, Product/1
  Add/1 -> Add1/1
  Demux/2 -> Add2/1
  Product3/1 -> Add1/2
  Add2/1 -> Add3/1
  Demux/1 -> Add/1
  Demux1/2 -> Product3/2, Product2/1  "q"
  Product/1 -> Add/2

== system UPQC_model/Shunt UPQC/Shuntkompensator/dq_Shunt/Entkopplungszelle43 ==
  In3 : Inport
  In4 : Inport  Port=2
  In1 : Inport  Port=3
  Add : Sum  Inputs=|+-
  Add1 : Sum  Inputs=|+-
  Add2 : Sum  Inputs=|++
  Add3 : Sum  Inputs=|+-
  Cos : Trigonometry  Operator=cos
  Demux : Demux  Outputs=2
  Demux1 : Demux  Outputs=2
  Mux : Mux  Inputs=2
  Product{,1..3} (4 alike) : Product
  Sin : Trigonometry
  Out2 : Outport
  wires:
  Product/1 -> Add/2
  Demux1/2 -> Product2/1, Product3/2  "q"
  Demux/1 -> Add/1
  Add2/1 -> Add3/1
  Product3/1 -> Add1/2
  Demux/2 -> Add2/1
  Add/1 -> Add1/1
  Cos/1 -> Product/1, Product2/2
  Sin/1 -> Product3/1, Product1/2
  In3/1 -> Demux/1  "vdqmit"
  Product2/1 -> Add3/2
  Product1/1 -> Add2/2
  Add1/1 -> Mux/1
  Add3/1 -> Mux/2
  In4/1 -> Cos/1, Sin/1  "theta"
  In1/1 -> Demux1/1  "dq"
  Demux1/1 -> Product/2, Product1/1  "d"
  Mux/1 -> Out2/1

== system UPQC_model/Shunt UPQC/Shuntkompensator/dq_Shunt/Entkopplungszelle44 ==
  In3 : Inport
  In4 : Inport  Port=2
  In1 : Inport  Port=3
  Add : Sum  Inputs=|+-
  Add1 : Sum  Inputs=|+-
  Add2 : Sum  Inputs=|++
  Add3 : Sum  Inputs=|+-
  Cos : Trigonometry  Operator=cos
  Demux : Demux  Outputs=2
  Demux1 : Demux  Outputs=2
  Mux : Mux  Inputs=2
  Product{,1..3} (4 alike) : Product
  Sin : Trigonometry
  Out2 : Outport
  wires:
  Product/1 -> Add/2
  Demux1/2 -> Product2/1, Product3/2  "q"
  Demux/1 -> Add/1
  Add2/1 -> Add3/1
  Product3/1 -> Add1/2
  Demux/2 -> Add2/1
  Add/1 -> Add1/1
  Cos/1 -> Product/1, Product2/2
  Sin/1 -> Product3/1, Product1/2
  In3/1 -> Demux/1  "vdqmit"
  Product2/1 -> Add3/2
  Product1/1 -> Add2/2
  Add1/1 -> Mux/1
  Add3/1 -> Mux/2
  In4/1 -> Cos/1, Sin/1  "theta"
  In1/1 -> Demux1/1  "dq"
  Demux1/1 -> Product/2, Product1/1  "d"
  Mux/1 -> Out2/1

== system UPQC_model/Shunt UPQC/Shuntkompensator/dq_Shunt/Entkopplungszelle45 ==
  In3 : Inport
  In4 : Inport  Port=2
  In1 : Inport  Port=3
  Add : Sum  Inputs=|+-
  Add1 : Sum  Inputs=|+-
  Add2 : Sum  Inputs=|++
  Add3 : Sum  Inputs=|+-
  Cos : Trigonometry  Operator=cos
  Demux : Demux  Outputs=2
  Demux1 : Demux  Outputs=2
  Mux : Mux  Inputs=2
  Product{,1..3} (4 alike) : Product
  Sin : Trigonometry
  Out2 : Outport
  wires:
  Product/1 -> Add/2
  Demux1/2 -> Product2/1, Product3/2  "q"
  Demux/1 -> Add/1
  Add2/1 -> Add3/1
  Product3/1 -> Add1/2
  Demux/2 -> Add2/1
  Add/1 -> Add1/1
  Cos/1 -> Product/1, Product2/2
  Sin/1 -> Product3/1, Product1/2
  In3/1 -> Demux/1  "vdqmit"
  Product2/1 -> Add3/2
  Product1/1 -> Add2/2
  Add1/1 -> Mux/1
  Add3/1 -> Mux/2
  In4/1 -> Cos/1, Sin/1  "theta"
  In1/1 -> Demux1/1  "dq"
  Demux1/1 -> Product/2, Product1/1  "d"
  Mux/1 -> Out2/1
